simulink model "C_identification"  (R2018b)
settings: Solver=FixedStepAuto  StartTime=0.0  StopTime=100  FixedStep=0.001  RelTol=1e-3
InitFcn:
  | Param
values from neighbouring files (symbols this model uses):
  tau = R*C    [C_id.m]    (also in Get_Square_Error.m = R*x; Identification.m; Minimization.m = 0)
settings Model: Creator=alessandrosebastianelli  LastModifiedBy=alessandrosebastianelli

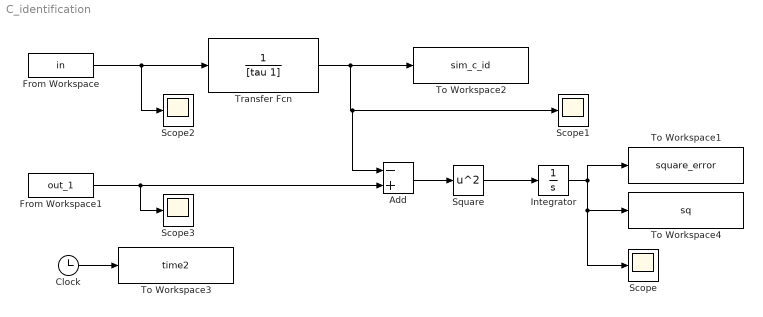
== system C_identification ==
  Add : Sum  Inputs=-+
  Clock : Clock
  From Workspace : FromWorkspace  VariableName=in  SampleTime=0
  From Workspace1 : FromWorkspace  VariableName=out_1  SampleTime=0
  Integrator : Integrator
  Scope{,1..3} (4 alike) : Scope
  Square : Math  Operator=square  SaturateOnIntegerOverflow=on
  To Workspace1 : ToWorkspace  VariableName=square_error  SampleTime=-1
      settings: Save2DSignal=2-D array (concatenate along first dimension)
  To Workspace2 : ToWorkspace  VariableName=sim_c_id  SampleTime=-1
      settings: Save2DSignal=2-D array (concatenate along first dimension)
  To Workspace3 : ToWorkspace  VariableName=time2  SampleTime=-1
      settings: Save2DSignal=2-D array (concatenate along first dimension)
  To Workspace4 : ToWorkspace  VariableName=sq  SampleTime=-1
      settings: Save2DSignal=2-D array (concatenate along first dimension)
  Transfer Fcn : TransferFcn  Denominator=[tau 1]  AbsoluteTolerance=-1
  wires:
  From Workspace/1 -> Transfer Fcn/1, Scope2/1
  From Workspace1/1 -> Scope3/1, Add/2
  Add/1 -> Square/1
  Square/1 -> Integrator/1
  Integrator/1 -> To Workspace4/1, Scope/1, To Workspace1/1
  Clock/1 -> To Workspace3/1
  Transfer Fcn/1 -> Add/1, Scope1/1, To Workspace2/1
